simulink model "TLBO_2023"  (R2023b)
settings: Solver=ode45  StartTime=0.0  StopTime=6  MaxStep=1e-4  RelTol=1e-3  EnableMultiTasking=on
PreLoadFcn:
  | Ts_Power=1e-6;
  | Ts_Control=100e-6;
InitFcn:
  | Ts_Power=1e-6;
  | Ts_Control=100e-6;
  | Rtrans=0.142;
  | Xtrans=0.12e-6;
undefined symbols (not defined in the file): DiscIntNeverNeededParam, Ion, Lithium, sigbuilder_block
libraries: dspfdesign x80, spsSeriesRLCBranchLib x52, spsCurrentMeasurementLib x20, spsMeanLib x20, spsIdealSwitchLib x16, spsVoltageMeasurementLib x16, slpidlib x15, spsMosfetLib x14, dspindex x12, spsPWMGeneratorDCDCLib x10, spsGroundLib x10, spsBatteryLib x4
(part 2 of 4)

== system TLBO_2023/DC Load 1_2 ==
  note: DC Load Control
  1 : dspfdesign/Analog Filter Design  method=Butterworth  filttype=Lowpass  N=8  Wlo=pi*50  Whi=80  Rp=2  Rs=40
  2 : dspfdesign/Analog Filter Design  method=Butterworth  filttype=Lowpass  N=8  Wlo=pi*50  Whi=80  Rp=2  Rs=40
  Current Measurement3 : spsCurrentMeasurementLib/Current Measurement  PhasorSimulation=off  OutputType=Complex  PSBequivalent=0
  Demux : Demux
  Ideal Switch{,1..3} (4 alike) : spsIdealSwitchLib/Ideal Switch  Ron=0.001  Lon=0  IC=0  Rs=1e5  Cs=inf  Measurements=off
  Load Control : Subsystem  Tag=STV Subsys  LoadFcn=sigbuilder_block('load');  StartFcn=sigbuilder_block('start');  StopFcn=sigbuilder_block('stop');  ClipboardFcn=sigbuilder_block('clipboard');  mask(Sigbuilder block){tuvar=[0:10]}
      mask help: Sigbuilder GUI
      mask init:
      | if ~strcmp(get_param(bdroot(gcbh),'SimulationStatus'),'stopped') tuvar = sigbuilder_block('maskInit'); end
      settings: CopyFcn=sigbuilder_block('copy');  DeleteFcn=sigbuilder_block('delete');  ModelCloseFcn=sigbuilder_block('modelClose');  PreSaveFcn=sigbuilder_block('preSave');  PauseFcn=sigbuilder_block('pause')  ContinueFcn=sigbuilder_block('continue')  NameChangeFcn=sigbuilder_block('namechange');  OpenFcn=sigbuilder_block('open',[5.4 30 1141.2 522.6 ]);  CloseFcn=sigbuilder_block('close');
      mask Display: plot(0, 0, 100, 100,[2, 2, 32, 32, 2], [68, 8, 8, 68, 68],[32, 2], [38, 38], [32, 19, 2],[53, 60, 44], [32, 17, 17, 2],[16, 16, 31, 31]);txt = getActiveGroup(gcbh);text(2, 100, txt,'verticalAlignment', 'top');
  Mux3 : Mux
  Product : Product
  Scope1 : Scope  NumInputPorts=2
  Series RLC Branch5 : spsSeriesRLCBranchLib/Series RLC Branch  LConnTagsString=__new0  RConnTagsString=__new0  BranchType=R  Resistance=5  Inductance=1e-3  SetiL0=off  InitialCurrent=0  Capacitance=1000e-6  Setx0=off  InitialVoltage=0  Measurements=None
  Series RLC Branch6 : spsSeriesRLCBranchLib/Series RLC Branch  LConnTagsString=__new0  RConnTagsString=__new0  BranchType=R  Resistance=50  Inductance=1e-3  SetiL0=off  InitialCurrent=0  Capacitance=1000e-6  Setx0=off  InitialVoltage=0  Measurements=None
  Series RLC Branch7 : spsSeriesRLCBranchLib/Series RLC Branch  LConnTagsString=__new0  RConnTagsString=__new0  BranchType=R  Resistance=11.5  Inductance=1e-3  SetiL0=off  InitialCurrent=0  Capacitance=1000e-6  Setx0=off  InitialVoltage=0  Measurements=None
  Series RLC Branch8 : spsSeriesRLCBranchLib/Series RLC Branch  LConnTagsString=__new0  RConnTagsString=__new0  BranchType=R  Resistance=11.5  Inductance=1e-3  SetiL0=off  InitialCurrent=0  Capacitance=1000e-6  Setx0=off  InitialVoltage=0  Measurements=None
  Series RLC Branch9 : spsSeriesRLCBranchLib/Series RLC Branch  LConnTagsString=__new0  RConnTagsString=__new0  BranchType=R  Resistance=11.5  Inductance=1e-3  SetiL0=off  InitialCurrent=0  Capacitance=1000e-6  Setx0=off  InitialVoltage=0  Measurements=None
  Voltage Measurement2 : spsVoltageMeasurementLib/Voltage Measurement  PhasorSimulation=off  OutputType=Complex  PSBequivalent=0
  + : PMIOPort  Side=Left
  - : PMIOPort  Port=2  Side=Right
  tag scope: I_L2=global, P_L2=global, V_L2=global
  wires:
  Product/1 -> [P_L2]
  Mux3/1 -> Demux/1
  Load Control/1(S1) -> Mux3/1
  Load Control/2(S2) -> Mux3/2
  Load Control/4(S4) -> Mux3/4
  Voltage Measurement2/1 -> 1/1
  Current Measurement3/1 -> 2/1
  Load Control/3(S3) -> Mux3/3
  Demux/2 -> Ideal Switch1/1  "S3"
  Demux/4 -> Ideal Switch3/1  "S5"
  Demux/1 -> Ideal Switch/1  "S2"
  Demux/3 -> Ideal Switch2/1  "S4"
  1/1 -> Scope1/2, [V_L2], Product/2  "Load Voltage"
  2/1 -> Scope1/1, [I_L2], Product/1  "Load Current"
  connections:
  +/RConn1 -- Current Measurement3/LConn1
  Ideal Switch/RConn1 -- Series RLC Branch6/LConn1
  Ideal Switch2/RConn1 -- Series RLC Branch8/LConn1
  Ideal Switch3/RConn1 -- Series RLC Branch9/LConn1
  Ideal Switch1/RConn1 -- Series RLC Branch7/LConn1
  -/RConn1 -- Series RLC Branch7/RConn1 -- Series RLC Branch8/RConn1 -- Series RLC Branch9/RConn1 -- Series RLC Branch6/RConn1 -- Series RLC Branch5/RConn1 -- Voltage Measurement2/LConn2
  Series RLC Branch5/LConn1 -- Ideal Switch2/LConn1 -- Ideal Switch3/LConn1 -- Ideal Switch1/LConn1 -- Ideal Switch/LConn1 -- Voltage Measurement2/LConn1 -- Current Measurement3/RConn1

== system TLBO_2023/DC Load 1_4 ==
  note: DC Load Control
  note: Maximum Load Power = 230W
  1 : dspfdesign/Analog Filter Design  method=Butterworth  filttype=Lowpass  N=8  Wlo=pi*50  Whi=80  Rp=2  Rs=40
  2 : dspfdesign/Analog Filter Design  method=Butterworth  filttype=Lowpass  N=8  Wlo=pi*50  Whi=80  Rp=2  Rs=40
  Current Measurement3 : spsCurrentMeasurementLib/Current Measurement  PhasorSimulation=off  OutputType=Complex  PSBequivalent=0
  Demux : Demux
  Ideal Switch{,1..3} (4 alike) : spsIdealSwitchLib/Ideal Switch  Ron=0.001  Lon=0  IC=0  Rs=1e5  Cs=inf  Measurements=off
  Load Control : Subsystem  Tag=STV Subsys  LoadFcn=sigbuilder_block('load');  StartFcn=sigbuilder_block('start');  StopFcn=sigbuilder_block('stop');  ClipboardFcn=sigbuilder_block('clipboard');  mask(Sigbuilder block){tuvar=[0:10]}
      mask help: Sigbuilder GUI
      mask init:
      | if ~strcmp(get_param(bdroot(gcbh),'SimulationStatus'),'stopped') tuvar = sigbuilder_block('maskInit'); end
      settings: CopyFcn=sigbuilder_block('copy');  DeleteFcn=sigbuilder_block('delete');  ModelCloseFcn=sigbuilder_block('modelClose');  PreSaveFcn=sigbuilder_block('preSave');  PauseFcn=sigbuilder_block('pause')  ContinueFcn=sigbuilder_block('continue')  NameChangeFcn=sigbuilder_block('namechange');  OpenFcn=sigbuilder_block('open',[5.4 30 1141.2 522.6 ]);  CloseFcn=sigbuilder_block('close');
      mask Display: plot(0, 0, 100, 100,[2, 2, 32, 32, 2], [68, 8, 8, 68, 68],[32, 2], [38, 38], [32, 19, 2],[53, 60, 44], [32, 17, 17, 2],[16, 16, 31, 31]);txt = getActiveGroup(gcbh);text(2, 100, txt,'verticalAlignment', 'top');
  Mux3 : Mux
  Product : Product
  Scope1 : Scope  NumInputPorts=2
  Series RLC Branch5 : spsSeriesRLCBranchLib/Series RLC Branch  LConnTagsString=__new0  RConnTagsString=__new0  BranchType=R  Resistance=5  Inductance=1e-3  SetiL0=off  InitialCurrent=0  Capacitance=1000e-6  Setx0=off  InitialVoltage=0  Measurements=None
  Series RLC Branch{6..9} (4 alike) : spsSeriesRLCBranchLib/Series RLC Branch  LConnTagsString=__new0  RConnTagsString=__new0  BranchType=R  Resistance=50  Inductance=1e-3  SetiL0=off  InitialCurrent=0  Capacitance=1000e-6  Setx0=off  InitialVoltage=0  Measurements=None
  Voltage Measurement2 : spsVoltageMeasurementLib/Voltage Measurement  PhasorSimulation=off  OutputType=Complex  PSBequivalent=0
  + : PMIOPort  Side=Left
  - : PMIOPort  Port=2  Side=Left
  tag scope: I_L1=global, P_L1=global, V_L1=global
  wires:
  Demux/3 -> Ideal Switch2/1  "S4"
  Demux/1 -> Ideal Switch/1  "S2"
  Demux/4 -> Ideal Switch3/1  "S5"
  Demux/2 -> Ideal Switch1/1  "S3"
  Load Control/3(S3) -> Mux3/3
  Current Measurement3/1 -> 2/1
  1/1 -> [V_L1], Product/2, Scope1/2  "Load Voltage"
  Voltage Measurement2/1 -> 1/1
  2/1 -> [I_L1], Product/1, Scope1/1  "Load Current"
  Load Control/4(S4) -> Mux3/4
  Load Control/2(S2) -> Mux3/2
  Load Control/1(S1) -> Mux3/1
  Mux3/1 -> Demux/1
  Product/1 -> [P_L1]
  connections:
  Ideal Switch2/LConn1 -- Ideal Switch3/LConn1 -- Ideal Switch1/LConn1 -- Ideal Switch/LConn1 -- Series RLC Branch5/LConn1 -- Current Measurement3/RConn1 -- Voltage Measurement2/LConn1
  Series RLC Branch7/RConn1 -- Series RLC Branch9/RConn1 -- Series RLC Branch8/RConn1 -- Series RLC Branch6/RConn1 -- Series RLC Branch5/RConn1 -- -/RConn1 -- Voltage Measurement2/LConn2
  Ideal Switch1/RConn1 -- Series RLC Branch7/LConn1
  Ideal Switch3/RConn1 -- Series RLC Branch9/LConn1
  Ideal Switch2/RConn1 -- Series RLC Branch8/LConn1
  Ideal Switch/RConn1 -- Series RLC Branch6/LConn1
  +/RConn1 -- Current Measurement3/LConn1

== system TLBO_2023/DC Load 2_3 ==
  note: DC Load Control
  note: Maximum Load Power = 230W
  1 : dspfdesign/Analog Filter Design  method=Butterworth  filttype=Lowpass  N=8  Wlo=pi*50  Whi=80  Rp=2  Rs=40
  2 : dspfdesign/Analog Filter Design  method=Butterworth  filttype=Lowpass  N=8  Wlo=pi*50  Whi=80  Rp=2  Rs=40
  Current Measurement3 : spsCurrentMeasurementLib/Current Measurement  PhasorSimulation=off  OutputType=Complex  PSBequivalent=0
  Demux : Demux
  Ideal Switch{,1..3} (4 alike) : spsIdealSwitchLib/Ideal Switch  Ron=0.001  Lon=0  IC=0  Rs=1e5  Cs=inf  Measurements=off
  Load Control : Subsystem  Tag=STV Subsys  LoadFcn=sigbuilder_block('load');  StartFcn=sigbuilder_block('start');  StopFcn=sigbuilder_block('stop');  ClipboardFcn=sigbuilder_block('clipboard');  mask(Sigbuilder block){tuvar=[0:10]}
      mask help: Sigbuilder GUI
      mask init:
      | if ~strcmp(get_param(bdroot(gcbh),'SimulationStatus'),'stopped') tuvar = sigbuilder_block('maskInit'); end
      settings: CopyFcn=sigbuilder_block('copy');  DeleteFcn=sigbuilder_block('delete');  ModelCloseFcn=sigbuilder_block('modelClose');  PreSaveFcn=sigbuilder_block('preSave');  PauseFcn=sigbuilder_block('pause')  ContinueFcn=sigbuilder_block('continue')  NameChangeFcn=sigbuilder_block('namechange');  OpenFcn=sigbuilder_block('open',[5.4 30 1141.2 522.6 ]);  CloseFcn=sigbuilder_block('close');
      mask Display: plot(0, 0, 100, 100,[2, 2, 32, 32, 2], [68, 8, 8, 68, 68],[32, 2], [38, 38], [32, 19, 2],[53, 60, 44], [32, 17, 17, 2],[16, 16, 31, 31]);txt = getActiveGroup(gcbh);text(2, 100, txt,'verticalAlignment', 'top');
  Mux3 : Mux
  Product : Product
  Scope1 : Scope  NumInputPorts=2
  Series RLC Branch{5,7..9} (4 alike) : spsSeriesRLCBranchLib/Series RLC Branch  LConnTagsString=__new0  RConnTagsString=__new0  BranchType=R  Resistance=5  Inductance=1e-3  SetiL0=off  InitialCurrent=0  Capacitance=1000e-6  Setx0=off  InitialVoltage=0  Measurements=None
  Series RLC Branch6 : spsSeriesRLCBranchLib/Series RLC Branch  LConnTagsString=__new0  RConnTagsString=__new0  BranchType=R  Resistance=50  Inductance=1e-3  SetiL0=off  InitialCurrent=0  Capacitance=1000e-6  Setx0=off  InitialVoltage=0  Measurements=None
  Voltage Measurement2 : spsVoltageMeasurementLib/Voltage Measurement  PhasorSimulation=off  OutputType=Complex  PSBequivalent=0
  + : PMIOPort  Side=Left
  - : PMIOPort  Port=2  Side=Left
  tag scope: I_L3=global, P_L3=global, V_L3=global
  wires:
  Demux/3 -> Ideal Switch2/1  "S4"
  Demux/1 -> Ideal Switch/1  "S2"
  Demux/4 -> Ideal Switch3/1  "S5"
  Demux/2 -> Ideal Switch1/1  "S3"
  Load Control/3(S3) -> Mux3/3
  Current Measurement3/1 -> 2/1
  Voltage Measurement2/1 -> 1/1
  Load Control/4(S4) -> Mux3/4
  Load Control/2(S2) -> Mux3/2
  Load Control/1(S1) -> Mux3/1
  Mux3/1 -> Demux/1
  Product/1 -> [P_L3]
  1/1 -> [V_L3], Product/2, Scope1/2  "Load Voltage"
  2/1 -> [I_L3], Product/1, Scope1/1  "Load Current"
  connections:
  Current Measurement3/RConn1 -- Voltage Measurement2/LConn1 -- Ideal Switch/LConn1 -- Ideal Switch1/LConn1 -- Ideal Switch3/LConn1 -- Ideal Switch2/LConn1 -- Series RLC Branch5/LConn1
  Voltage Measurement2/LConn2 -- Series RLC Branch5/RConn1 -- Series RLC Branch6/RConn1 -- Series RLC Branch9/RConn1 -- Series RLC Branch8/RConn1 -- Series RLC Branch7/RConn1 -- -/RConn1
  Ideal Switch1/RConn1 -- Series RLC Branch7/LConn1
  Ideal Switch3/RConn1 -- Series RLC Branch9/LConn1
  Ideal Switch2/RConn1 -- Series RLC Branch8/LConn1
  Ideal Switch/RConn1 -- Series RLC Branch6/LConn1
  +/RConn1 -- Current Measurement3/LConn1

== system TLBO_2023/DC Load 3_4 ==
  note: DC Load Control
  1 : dspfdesign/Analog Filter Design  method=Butterworth  filttype=Lowpass  N=8  Wlo=pi*50  Whi=80  Rp=2  Rs=40
  2 : dspfdesign/Analog Filter Design  method=Butterworth  filttype=Lowpass  N=8  Wlo=pi*50  Whi=80  Rp=2  Rs=40
  Current Measurement3 : spsCurrentMeasurementLib/Current Measurement  PhasorSimulation=off  OutputType=Complex  PSBequivalent=0
  Demux : Demux
  Ideal Switch{,1..3} (4 alike) : spsIdealSwitchLib/Ideal Switch  Ron=0.001  Lon=0  IC=0  Rs=1e5  Cs=inf  Measurements=off
  Load Control : Subsystem  Tag=STV Subsys  LoadFcn=sigbuilder_block('load');  StartFcn=sigbuilder_block('start');  StopFcn=sigbuilder_block('stop');  ClipboardFcn=sigbuilder_block('clipboard');  mask(Sigbuilder block){tuvar=[0:10]}
      mask help: Sigbuilder GUI
      mask init:
      | if ~strcmp(get_param(bdroot(gcbh),'SimulationStatus'),'stopped') tuvar = sigbuilder_block('maskInit'); end
      settings: CopyFcn=sigbuilder_block('copy');  DeleteFcn=sigbuilder_block('delete');  ModelCloseFcn=sigbuilder_block('modelClose');  PreSaveFcn=sigbuilder_block('preSave');  PauseFcn=sigbuilder_block('pause')  ContinueFcn=sigbuilder_block('continue')  NameChangeFcn=sigbuilder_block('namechange');  OpenFcn=sigbuilder_block('open',[5.4 30 1141.2 522.6 ]);  CloseFcn=sigbuilder_block('close');
      mask Display: plot(0, 0, 100, 100,[2, 2, 32, 32, 2], [68, 8, 8, 68, 68],[32, 2], [38, 38], [32, 19, 2],[53, 60, 44], [32, 17, 17, 2],[16, 16, 31, 31]);txt = getActiveGroup(gcbh);text(2, 100, txt,'verticalAlignment', 'top');
  Mux3 : Mux
  Product : Product
  Scope1 : Scope  NumInputPorts=2
  Series RLC Branch5 : spsSeriesRLCBranchLib/Series RLC Branch  LConnTagsString=__new0  RConnTagsString=__new0  BranchType=R  Resistance=5  Inductance=1e-3  SetiL0=off  InitialCurrent=0  Capacitance=1000e-6  Setx0=off  InitialVoltage=0  Measurements=None
  Series RLC Branch6 : spsSeriesRLCBranchLib/Series RLC Branch  LConnTagsString=__new0  RConnTagsString=__new0  BranchType=R  Resistance=50  Inductance=1e-3  SetiL0=off  InitialCurrent=0  Capacitance=1000e-6  Setx0=off  InitialVoltage=0  Measurements=None
  Series RLC Branch7 : spsSeriesRLCBranchLib/Series RLC Branch  LConnTagsString=__new0  RConnTagsString=__new0  BranchType=R  Resistance=11.5  Inductance=1e-3  SetiL0=off  InitialCurrent=0  Capacitance=1000e-6  Setx0=off  InitialVoltage=0  Measurements=None
  Series RLC Branch8 : spsSeriesRLCBranchLib/Series RLC Branch  LConnTagsString=__new0  RConnTagsString=__new0  BranchType=R  Resistance=11.5  Inductance=1e-3  SetiL0=off  InitialCurrent=0  Capacitance=1000e-6  Setx0=off  InitialVoltage=0  Measurements=None
  Series RLC Branch9 : spsSeriesRLCBranchLib/Series RLC Branch  LConnTagsString=__new0  RConnTagsString=__new0  BranchType=R  Resistance=11.5  Inductance=1e-3  SetiL0=off  InitialCurrent=0  Capacitance=1000e-6  Setx0=off  InitialVoltage=0  Measurements=None
  Voltage Measurement2 : spsVoltageMeasurementLib/Voltage Measurement  PhasorSimulation=off  OutputType=Complex  PSBequivalent=0
  + : PMIOPort  Side=Left
  - : PMIOPort  Port=2  Side=Right
  tag scope: I_L4=global, P_L4=global, V_L4=global
  wires:
  Product/1 -> [P_L4]
  Mux3/1 -> Demux/1
  Load Control/1(S1) -> Mux3/1
  Load Control/2(S2) -> Mux3/2
  Load Control/4(S4) -> Mux3/4
  Voltage Measurement2/1 -> 1/1
  Current Measurement3/1 -> 2/1
  Load Control/3(S3) -> Mux3/3
  Demux/2 -> Ideal Switch1/1  "S3"
  Demux/4 -> Ideal Switch3/1  "S5"
  Demux/1 -> Ideal Switch/1  "S2"
  Demux/3 -> Ideal Switch2/1  "S4"
  1/1 -> Scope1/2, [V_L4], Product/2  "Load Voltage"
  2/1 -> Scope1/1, [I_L4], Product/1  "Load Current"
  connections:
  +/RConn1 -- Current Measurement3/LConn1
  Ideal Switch/RConn1 -- Series RLC Branch6/LConn1
  Ideal Switch2/RConn1 -- Series RLC Branch8/LConn1
  Ideal Switch3/RConn1 -- Series RLC Branch9/LConn1
  Ideal Switch1/RConn1 -- Series RLC Branch7/LConn1
  -/RConn1 -- Series RLC Branch7/RConn1 -- Series RLC Branch8/RConn1 -- Series RLC Branch9/RConn1 -- Series RLC Branch6/RConn1 -- Series RLC Branch5/RConn1 -- Voltage Measurement2/LConn2
  Series RLC Branch5/LConn1 -- Ideal Switch2/LConn1 -- Ideal Switch3/LConn1 -- Ideal Switch1/LConn1 -- Ideal Switch/LConn1 -- Voltage Measurement2/LConn1 -- Current Measurement3/RConn1

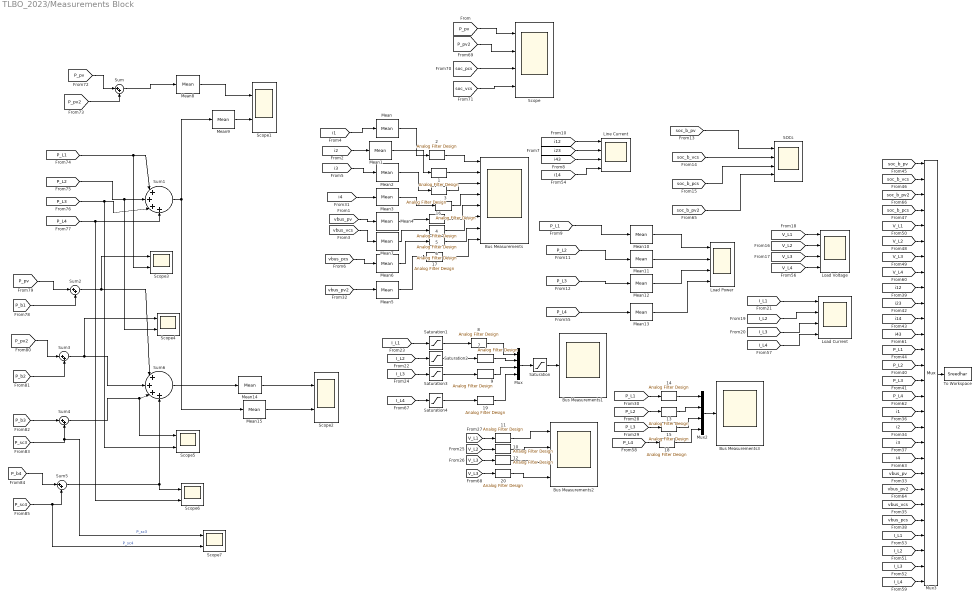
== system TLBO_2023/Measurements Block ==
  {1..20} (20 alike) : dspfdesign/Analog Filter Design  method=Butterworth  filttype=Lowpass  N=8  Wlo=pi*50  Whi=80  Rp=2  Rs=40
  Bus Measurements : Scope  NumInputPorts=8
  Bus Measurements1 : Scope
  Bus Measurements2 : Scope  NumInputPorts=4
  Bus Measurements3 : Scope
  Line Current : Scope  NumInputPorts=4
  Load Current : Scope  NumInputPorts=4
  Load Power : Scope  NumInputPorts=4
  Load Voltage : Scope  NumInputPorts=4
  Mean{,1..15} (16 alike) : spsMeanLib/Mean  Freq=10  Vinit=0  Ts=0
  Mux : Mux
  Mux2 : Mux
  Mux3 : Mux  Inputs=28
  SOCs : Scope  NumInputPorts=4
  Saturation{,1..4} (5 alike) : Saturate  UpperLimit=50  LowerLimit=0
  Scope : Scope  NumInputPorts=4
  Scope{1..7} (7 alike) : Scope  NumInputPorts=2
  Sum{,2..5} (5 alike) : Sum  Inputs=|++
  Sum1 : Sum  Inputs=|++++
  Sum6 : Sum  Inputs=|++++
  To Workspace : ToWorkspace  VariableName=Sreedhar  SampleTime=-1
  wires:
  [i12] -> Line Current/1
  [i23] -> Line Current/2
  [i43] -> Line Current/3
  [soc_b_pv] -> SOCs/1
  [soc_b_vcs] -> SOCs/2
  [soc_b_pcs] -> SOCs/3
  [V_L1] -> Load Voltage/1
  [V_L2] -> Load Voltage/2
  [V_L3] -> Load Voltage/3
  [I_L1] -> Load Current/1
  [I_L2] -> Load Current/2
  [I_L3] -> Load Current/3
  2/1 -> Bus Measurements/1
  1/1 -> Bus Measurements/2
  3/1 -> Bus Measurements/3
  9/1 -> Mux/3
  7/1 -> Mux/2
  8/1 -> Mux/1
  11/1 -> Bus Measurements2/1
  [V_L1] -> 11/1
  [V_L2] -> 10/1
  [V_L3] -> 12/1
  10/1 -> Bus Measurements2/2
  12/1 -> Bus Measurements2/3
  Mux2/1 -> Bus Measurements3/1
  14/1 -> Mux2/1
  13/1 -> Mux2/2
  15/1 -> Mux2/3
  [P_L1] -> 14/1
  [P_L2] -> 13/1
  [P_L3] -> 15/1
  Mux/1 -> Saturation/1
  Saturation/1 -> Bus Measurements1/1
  [I_L1] -> Saturation1/1
  Saturation1/1 -> 8/1
  [I_L2] -> Saturation2/1
  Saturation2/1 -> 7/1
  [I_L3] -> Saturation3/1
  Saturation3/1 -> 9/1
  Mux3/1 -> To Workspace/1
  [V_L1] -> Mux3/5
  [soc_b_pcs] -> Mux3/4
  [soc_b_vcs] -> Mux3/2
  [soc_b_pv] -> Mux3/1
  6/1 -> Bus Measurements/7
  5/1 -> Bus Measurements/6
  4/1 -> Bus Measurements/5
  16/1 -> Bus Measurements/4
  17/1 -> Bus Measurements/8
  [i14] -> Line Current/4
  [V_L4] -> Load Voltage/4
  [I_L4] -> Load Current/4
  [P_L4] -> 18/1
  18/1 -> Mux2/4
  [V_L2] -> Mux3/6
  [V_L3] -> Mux3/7
  [V_L4] -> Mux3/8
  [i12] -> Mux3/9
  [i23] -> Mux3/10
  [i14] -> Mux3/11
  [i43] -> Mux3/12
  [P_L1] -> Mux3/13
  [P_L2] -> Mux3/14
  [P_L3] -> Mux3/15
  [P_L4] -> Mux3/16
  [i1] -> Mux3/17
  [i2] -> Mux3/18
  [i3] -> Mux3/19
  [i4] -> Mux3/20
  [vbus_pv] -> Mux3/21
  [vbus_pv2] -> Mux3/22
  [vbus_vcs] -> Mux3/23
  [vbus_pcs] -> Mux3/24
  [I_L1] -> Mux3/25
  [I_L2] -> Mux3/26
  [I_L3] -> Mux3/27
  [I_L4] -> Mux3/28
  [soc_b_pv2] -> SOCs/4
  [soc_b_pv2] -> Mux3/3
  [I_L4] -> Saturation4/1
  Saturation4/1 -> 19/1
  19/1 -> Mux/4
  [V_L3] -> 20/1
  20/1 -> Bus Measurements2/4
  [P_pv] -> Scope/1
  [P_pv2] -> Scope/2
  [soc_pcs] -> Scope/3
  [soc_vcs] -> Scope/4
  [P_pv] -> Sum/1
  [P_pv2] -> Sum/2
  [P_L1] -> Scope3/2, Sum1/1
  [P_L2] -> Scope4/2, Sum1/2
  [P_L3] -> Scope5/2, Sum1/3
  [P_L4] -> Scope6/2, Sum1/4
  Sum1/1 -> Mean9/1, Mean15/1
  [P_pv] -> Sum2/1
  [P_b1] -> Sum2/2
  [P_pv2] -> Sum3/1
  [P_b2] -> Sum3/2
  [P_b3] -> Sum4/1
  [P_sc3] -> Scope7/1, Sum4/2  "P_sc3"
  [P_b4] -> Sum5/1
  [P_sc4] -> Scope7/2, Sum5/2  "P_sc4"
  Sum2/1 -> Scope3/1, Sum6/1
  Sum3/1 -> Scope4/1, Sum6/2
  Sum4/1 -> Scope5/1, Sum6/3
  Sum5/1 -> Sum6/4, Scope6/1
  Sum6/1 -> Mean14/1
  [i1] -> Mean/1
  Mean/1 -> 2/1
  [i2] -> Mean1/1
  Mean1/1 -> 1/1
  [i3] -> Mean2/1
  Mean2/1 -> 3/1
  [i4] -> Mean3/1
  Mean3/1 -> 16/1
  [vbus_pv] -> Mean4/1
  Mean4/1 -> 4/1
  [vbus_pv2] -> Mean5/1
  Mean5/1 -> 17/1
  [vbus_pcs] -> Mean6/1
  Mean6/1 -> 6/1
  [vbus_vcs] -> Mean7/1
  Mean7/1 -> 5/1
  Sum/1 -> Mean8/1
  Mean8/1 -> Scope1/1
  Mean9/1 -> Scope1/2
  [P_L1] -> Mean10/1
  Mean10/1 -> Load Power/1
  [P_L2] -> Mean11/1
  Mean11/1 -> Load Power/2
  [P_L3] -> Mean12/1
  Mean12/1 -> Load Power/3
  [P_L4] -> Mean13/1
  Mean13/1 -> Load Power/4
  Mean14/1 -> Scope2/1
  Mean15/1 -> Scope2/2

== system TLBO_2023/Source1 ==
  Battery Storage : Subsystem
  P_b : Display
      settings: Format=bank  Decimation=1000
  P_pv : Display
      settings: Format=bank  Decimation=1000
  R1 : spsSeriesRLCBranchLib/Series RLC Branch  LConnTagsString=__new0  RConnTagsString=__new0  BranchType=R  Resistance=0.2  Inductance=1e-3  SetiL0=off  InitialCurrent=0  Capacitance=220e-6  Setx0=off  InitialVoltage=0  Measurements=None
  R2 : spsSeriesRLCBranchLib/Series RLC Branch  LConnTagsString=__new0  RConnTagsString=__new0  BranchType=R  Resistance=0.2  Inductance=1e-3  SetiL0=off  InitialCurrent=0  Capacitance=220e-6  Setx0=off  InitialVoltage=0  Measurements=None
  Rooftop Solar System : Subsystem
  SOC_b : Display
      settings: Format=bank  Decimation=1000
  + : PMIOPort  Side=Right
  - : PMIOPort  Port=2  Side=Right
  tag scope: P_b1=global, P_pv=global, soc_pv=global
  wires:
  Battery Storage/2(Power) -> [P_b1], P_b/1
  Battery Storage/1(SOC) -> [soc_pv], SOC_b/1
  Rooftop Solar System/1(Power) -> [P_pv], P_pv/1
  connections:
  R1/LConn1 -- +/RConn1 -- R2/LConn1
  R1/RConn1 -- Rooftop Solar System/RConn1
  R2/RConn1 -- Battery Storage/RConn1
  Rooftop Solar System/RConn2 -- -/RConn1 -- Battery Storage/RConn2

== system TLBO_2023/Source2 ==
  Battery Storage : Subsystem
  P_b : Display
      settings: Format=bank  Decimation=1000
  P_pv : Display
      settings: Format=bank  Decimation=1000
  R1 : spsSeriesRLCBranchLib/Series RLC Branch  LConnTagsString=__new0  RConnTagsString=__new0  BranchType=R  Resistance=0.2  Inductance=1e-3  SetiL0=off  InitialCurrent=0  Capacitance=220e-6  Setx0=off  InitialVoltage=0  Measurements=None
  R2 : spsSeriesRLCBranchLib/Series RLC Branch  LConnTagsString=__new0  RConnTagsString=__new0  BranchType=R  Resistance=0.2  Inductance=1e-3  SetiL0=off  InitialCurrent=0  Capacitance=220e-6  Setx0=off  InitialVoltage=0  Measurements=None
  Rooftop Solar System : Subsystem
  SOC_b : Display
      settings: Format=bank  Decimation=1000
  + : PMIOPort  Side=Right
  - : PMIOPort  Port=2  Side=Right
  tag scope: P_b2=global, P_pv2=global, soc_pv2=global
  wires:
  Battery Storage/2(Power) -> [P_b2], P_b/1
  Battery Storage/1(SOC) -> [soc_pv2], SOC_b/1
  Rooftop Solar System/1(Power) -> [P_pv2], P_pv/1
  connections:
  R1/LConn1 -- +/RConn1 -- R2/LConn1
  R1/RConn1 -- Rooftop Solar System/RConn1
  R2/RConn1 -- Battery Storage/RConn1
  Rooftop Solar System/RConn2 -- -/RConn1 -- Battery Storage/RConn2

== system TLBO_2023/Source3 ==
  Battery Storage : Subsystem
  P_pcs : Display
      settings: Format=bank  Decimation=1000
  P_sc_pcs : Display
      settings: Format=bank  Decimation=1000
  R1 : spsSeriesRLCBranchLib/Series RLC Branch  LConnTagsString=__new0  RConnTagsString=__new0  BranchType=R  Resistance=0.2  Inductance=1e-3  SetiL0=off  InitialCurrent=0  Capacitance=220e-6  Setx0=off  InitialVoltage=0  Measurements=None
  R2 : spsSeriesRLCBranchLib/Series RLC Branch  LConnTagsString=__new0  RConnTagsString=__new0  BranchType=R  Resistance=0.2  Inductance=1e-3  SetiL0=off  InitialCurrent=0  Capacitance=220e-6  Setx0=off  InitialVoltage=0  Measurements=None
  SOC_pcs : Display
      settings: Format=bank  Decimation=1000
  SOC_sc_pcs : Display
      settings: Format=bank  Decimation=1000
  Scope : Scope  NumInputPorts=2
  Super Capacitor : Subsystem
  + : PMIOPort  Side=Right
  - : PMIOPort  Port=2  Side=Left
  tag scope: P_b3=global, P_sc3=global, soc_pcs=global, soc_sc_pcs=global
  wires:
  Battery Storage/1(SOC) -> SOC_pcs/1, [soc_pcs]
  Battery Storage/2(Power) -> [P_b3], P_pcs/1
  Super Capacitor/1(SOC) -> [soc_sc_pcs], Scope/1, SOC_sc_pcs/1
  Super Capacitor/2(Power) -> [P_sc3], Scope/2, P_sc_pcs/1
  connections:
  Battery Storage/RConn2 -- Super Capacitor/RConn2 -- -/RConn1
  R2/RConn1 -- Battery Storage/RConn1
  R2/LConn1 -- R1/LConn1 -- +/RConn1
  Super Capacitor/RConn1 -- R1/RConn1

== system TLBO_2023/Source4 ==
  Battery Storage : Subsystem
  P_sc_vcs : Display
      settings: Format=bank  Decimation=1000
  P_vcs : Display
      settings: Format=bank  Decimation=1000
  R1 : spsSeriesRLCBranchLib/Series RLC Branch  LConnTagsString=__new0  RConnTagsString=__new0  BranchType=R  Resistance=0.2  Inductance=1e-3  SetiL0=off  InitialCurrent=0  Capacitance=220e-6  Setx0=off  InitialVoltage=0  Measurements=None
  R2 : spsSeriesRLCBranchLib/Series RLC Branch  LConnTagsString=__new0  RConnTagsString=__new0  BranchType=R  Resistance=0.2  Inductance=1e-3  SetiL0=off  InitialCurrent=0  Capacitance=220e-6  Setx0=off  InitialVoltage=0  Measurements=None
  SOC_sc_vcs : Display
      settings: Format=bank  Decimation=1000
  SOC_vcs : Display
      settings: Format=bank  Decimation=1000
  Scope5 : Scope  NumInputPorts=2
  Super Capacitor : Subsystem
  + : PMIOPort  Side=Right
  - : PMIOPort  Port=2  Side=Right
  tag scope: P_b4=global, P_sc4=global, Soc_sc_vcs=global, soc_vcs=global
  wires:
  Battery Storage/2(Power) -> [P_b4], P_vcs/1
  Battery Storage/1(SOC) -> [soc_vcs], SOC_vcs/1
  Super Capacitor/1(SOC) -> [Soc_sc_vcs], Scope5/1, SOC_sc_vcs/1
  Super Capacitor/2(Power) -> [P_sc4], Scope5/2, P_sc_vcs/1
  connections:
  +/RConn1 -- R1/LConn1 -- R2/LConn1
  R2/RConn1 -- Battery Storage/RConn1
  Battery Storage/RConn2 -- Super Capacitor/RConn2 -- -/RConn1
  Super Capacitor/RConn1 -- R1/RConn1

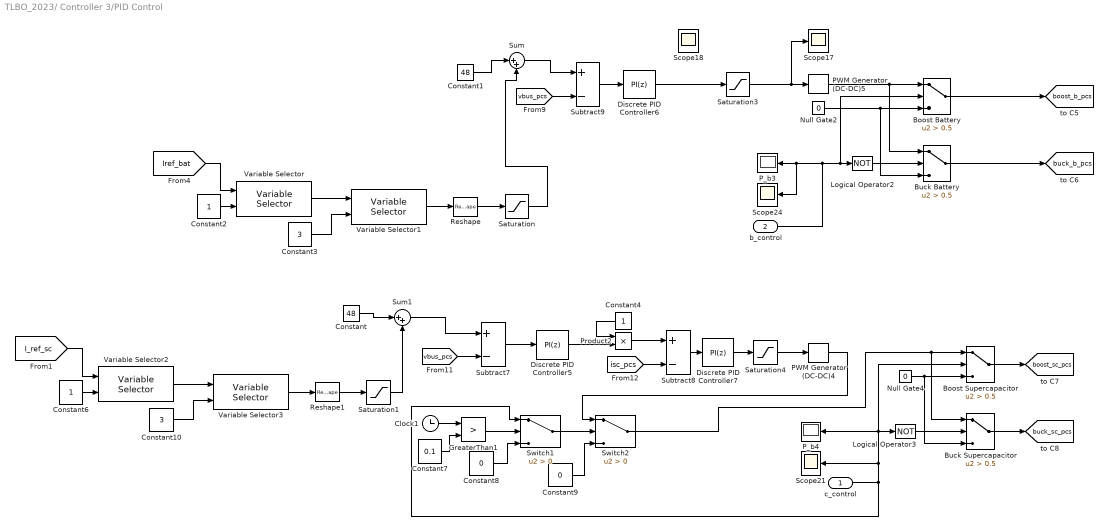
== system TLBO_2023/ Controller 3/PID Control ==
  c_control : Inport
  b_control : Inport  Port=2
  Boost Battery : Switch  Criteria=u2 > Threshold  Threshold=0.5  SaturateOnIntegerOverflow=off  InputSameDT=off
  Boost Supercapacitor : Switch  Criteria=u2 > Threshold  Threshold=0.5  SaturateOnIntegerOverflow=off  InputSameDT=off
  Buck Battery : Switch  Criteria=u2 > Threshold  Threshold=0.5  SaturateOnIntegerOverflow=off  InputSameDT=off
  Buck Supercapacitor : Switch  Criteria=u2 > Threshold  Threshold=0.5  SaturateOnIntegerOverflow=off  InputSameDT=off
  Clock1 : Clock
  Constant : Constant  Value=48
  Constant1 : Constant  Value=48
  Constant10 : Constant  Value=3
  Constant2 : Constant
  Constant3 : Constant  Value=3
  Constant4 : Constant
  Constant6 : Constant
  Constant7 : Constant  Value=0.1
  Constant8 : Constant  Value=0
  Constant9 : Constant  Value=0
  Discrete PID Controller5 : slpidlib/PID Controller  Controller=PI  Form=Parallel  TimeDomain=Discrete-time  UseExternalTs=off  SampleTime=-1  IntegratorMethod=Forward Euler  FilterMethod=Forward Euler  ControllerParametersSource=internal  P=0  I=4  UseKiTs=off  D=1  N=100  UseFilter=on  TunerSelectOption=Transfer Function Based (PID Tuner App)  InitialConditionSource=internal  InitialConditionForIntegrator=0  InitialConditionForFilter=0  DifferentiatorICPrevScaledInput=0  ExternalReset=none  TrackingMode=off  Kt=1  LimitOutput=off  SatLimitsSource=internal  UpperSaturationLimit=inf  LowerSaturationLimit=-inf  LinearizeAsGain=off  AntiWindupMode=none  Kb=1  LimitIntegrator=off  UpperIntegratorSaturationLimit=inf  LowerIntegratorSaturationLimit=-inf  POutMin=[]  POutMax=[]  IOutMin=[]  IOutMax=[]  DOutMin=[]  DOutMax=[]  NOutMin=[]  NOutMax=[]  SumOutMin=[]  SumOutMax=[]  SaturationOutMin=[]  SaturationOutMax=[]  PParamMin=[]  PParamMax=[]  IParamMin=[]  IParamMax=[]  DParamMin=[]  DParamMax=[]  NParamMin=[]  NParamMax=[]  KbParamMin=[]  KbParamMax=[]  KtParamMin=[]  KtParamMax=[]  KbOutMin=[]  KbOutMax=[]  KtOutMin=[]  KtOutMax=[]  IntegratorOutMin=[]  IntegratorOutMax=[]  FilterOutMin=[]  FilterOutMax=[]  SumI1OutMin=[]  SumI1OutMax=[]  SumI2OutMin=[]  SumI2OutMax=[]  SumI3OutMin=[]  SumI3OutMax=[]  SumI4OutMin=[]  SumI4OutMax=[]  SumDOutMin=[]  SumDOutMax=[]  DifferentiatorOutMin=[]  DifferentiatorOutMax=[]  FilterDiffOutCoefMin=[]  FilterDiffOutCoefMax=[]  ReciprocalOutMin=[]  ReciprocalOutMax=[]  SumDenOutMin=[]  SumDenOutMax=[]  SumNumOutMin=[]  SumNumOutMax=[]  DivideOutMin=[]  DivideOutMax=[]  UdiffTsProdOutMin=[]  UdiffTsProdOutMax=[]  NTsProdOutMin=[]  NTsProdOutMax=[]  UintegralTsProdOutMin=[]  UintegralTsProdOutMax=[]  UngainTsProdOutMin=[]  UngainTsProdOutMax=[]  ClampingZeroOutDataTypeStr=Inherit: Inherit via back propagation  ClampingZeroOutMin=[]  ClampingZeroOutMax=[]  FilterDenConstantOutDataTypeStr=Inherit: Inherit via back propagation  FilterDenConstantOutMin=[]  FilterDenConstantOutMax=[]  PCopyOutDataTypeStr=Inherit: Inherit via back propagation  PCopyOutMin=[]  PCopyOutMax=[]  NCopyOutDataTypeStr=Inherit: Inherit via back propagation  NCopyOutMin=[]  NCopyOutMax=[]  IntegratorContinuousStateAttributes=''  IntegratorStateMustResolveToSignalObject=off  IntegratorRTWStateStorageClass=Auto  FilterContinuousStateAttributes=''  FilterStateMustResolveToSignalObject=off  FilterRTWStateStorageClass=Auto  ParallelPVariant=InternalParameters  IdealPVariant=Disabled  IVariant=InternalParameters  DVariant=Disabled  IntegratorVariant=Discrete  SatVariant=Disabled  AWVariant=Passthrough  PCopyVariant=Disabled  TRVariant=Disabled  FdbkBlocksVariant=Forward  IdealPFdbkVariant=Disabled  SatFdbkVariant=Disabled  DerivativeFilterVariant=Disabled  NVariant=Disabled  NCopyVariant=Disabled_SignalSpec  FilterICVariant=Disabled  IntegratorICVariant=InternalICs  ExternalResetVariant=Disabled  TRSumVariant=Passthrough  SumFdbkVariant=Disabled  SumVariant=Sum_PI  TsampFilterVariant=InternalTs  TsampNgainVariant=Passthrough  TsampIntegralVariant=Disabled_SignalSpec  ExternalSaturationOutDataTypeStr=Inherit: Same as second input
  Discrete PID Controller6 : slpidlib/PID Controller  Controller=PI  Form=Parallel  TimeDomain=Discrete-time  UseExternalTs=off  SampleTime=-1  IntegratorMethod=Forward Euler  FilterMethod=Forward Euler  ControllerParametersSource=internal  P=0  I=1  UseKiTs=off  D=1  N=100  UseFilter=on  TunerSelectOption=Transfer Function Based (PID Tuner App)  InitialConditionSource=internal  InitialConditionForIntegrator=0  InitialConditionForFilter=0  DifferentiatorICPrevScaledInput=0  ExternalReset=none  TrackingMode=off  Kt=1  LimitOutput=off  SatLimitsSource=internal  UpperSaturationLimit=inf  LowerSaturationLimit=-inf  LinearizeAsGain=off  AntiWindupMode=none  Kb=1  LimitIntegrator=off  UpperIntegratorSaturationLimit=inf  LowerIntegratorSaturationLimit=-inf  POutMin=[]  POutMax=[]  IOutMin=[]  IOutMax=[]  DOutMin=[]  DOutMax=[]  NOutMin=[]  NOutMax=[]  SumOutMin=[]  SumOutMax=[]  SaturationOutMin=[]  SaturationOutMax=[]  PParamMin=[]  PParamMax=[]  IParamMin=[]  IParamMax=[]  DParamMin=[]  DParamMax=[]  NParamMin=[]  NParamMax=[]  KbParamMin=[]  KbParamMax=[]  KtParamMin=[]  KtParamMax=[]  KbOutMin=[]  KbOutMax=[]  KtOutMin=[]  KtOutMax=[]  IntegratorOutMin=[]  IntegratorOutMax=[]  FilterOutMin=[]  FilterOutMax=[]  SumI1OutMin=[]  SumI1OutMax=[]  SumI2OutMin=[]  SumI2OutMax=[]  SumI3OutMin=[]  SumI3OutMax=[]  SumI4OutMin=[]  SumI4OutMax=[]  SumDOutMin=[]  SumDOutMax=[]  DifferentiatorOutMin=[]  DifferentiatorOutMax=[]  FilterDiffOutCoefMin=[]  FilterDiffOutCoefMax=[]  ReciprocalOutMin=[]  ReciprocalOutMax=[]  SumDenOutMin=[]  SumDenOutMax=[]  SumNumOutMin=[]  SumNumOutMax=[]  DivideOutMin=[]  DivideOutMax=[]  UdiffTsProdOutMin=[]  UdiffTsProdOutMax=[]  NTsProdOutMin=[]  NTsProdOutMax=[]  UintegralTsProdOutMin=[]  UintegralTsProdOutMax=[]  UngainTsProdOutMin=[]  UngainTsProdOutMax=[]  ClampingZeroOutDataTypeStr=Inherit: Inherit via back propagation  ClampingZeroOutMin=[]  ClampingZeroOutMax=[]  FilterDenConstantOutDataTypeStr=Inherit: Inherit via back propagation  FilterDenConstantOutMin=[]  FilterDenConstantOutMax=[]  PCopyOutDataTypeStr=Inherit: Inherit via back propagation  PCopyOutMin=[]  PCopyOutMax=[]  NCopyOutDataTypeStr=Inherit: Inherit via back propagation  NCopyOutMin=[]  NCopyOutMax=[]  IntegratorContinuousStateAttributes=''  IntegratorStateMustResolveToSignalObject=off  IntegratorRTWStateStorageClass=Auto  FilterContinuousStateAttributes=''  FilterStateMustResolveToSignalObject=off  FilterRTWStateStorageClass=Auto  ParallelPVariant=InternalParameters  IdealPVariant=Disabled  IVariant=InternalParameters  DVariant=Disabled  IntegratorVariant=Discrete  SatVariant=Disabled  AWVariant=Passthrough  PCopyVariant=Disabled  TRVariant=Disabled  FdbkBlocksVariant=Forward  IdealPFdbkVariant=Disabled  SatFdbkVariant=Disabled  DerivativeFilterVariant=Disabled  NVariant=Disabled  NCopyVariant=Disabled_SignalSpec  FilterICVariant=Disabled  IntegratorICVariant=InternalICs  ExternalResetVariant=Disabled  TRSumVariant=Passthrough  SumFdbkVariant=Disabled  SumVariant=Sum_PI  TsampFilterVariant=InternalTs  TsampNgainVariant=Passthrough  TsampIntegralVariant=Disabled_SignalSpec  ExternalSaturationOutDataTypeStr=Inherit: Same as second input
  Discrete PID Controller7 : slpidlib/PID Controller  Controller=PI  Form=Parallel  TimeDomain=Discrete-time  UseExternalTs=off  SampleTime=-1  IntegratorMethod=Forward Euler  FilterMethod=Forward Euler  ControllerParametersSource=internal  P=0.2  I=4  UseKiTs=off  D=1  N=100  UseFilter=on  TunerSelectOption=Transfer Function Based (PID Tuner App)  InitialConditionSource=internal  InitialConditionForIntegrator=0  InitialConditionForFilter=0  DifferentiatorICPrevScaledInput=0  ExternalReset=none  TrackingMode=off  Kt=1  LimitOutput=off  SatLimitsSource=internal  UpperSaturationLimit=inf  LowerSaturationLimit=-inf  LinearizeAsGain=off  AntiWindupMode=none  Kb=1  LimitIntegrator=off  UpperIntegratorSaturationLimit=inf  LowerIntegratorSaturationLimit=-inf  POutMin=[]  POutMax=[]  IOutMin=[]  IOutMax=[]  DOutMin=[]  DOutMax=[]  NOutMin=[]  NOutMax=[]  SumOutMin=[]  SumOutMax=[]  SaturationOutMin=[]  SaturationOutMax=[]  PParamMin=[]  PParamMax=[]  IParamMin=[]  IParamMax=[]  DParamMin=[]  DParamMax=[]  NParamMin=[]  NParamMax=[]  KbParamMin=[]  KbParamMax=[]  KtParamMin=[]  KtParamMax=[]  KbOutMin=[]  KbOutMax=[]  KtOutMin=[]  KtOutMax=[]  IntegratorOutMin=[]  IntegratorOutMax=[]  FilterOutMin=[]  FilterOutMax=[]  SumI1OutMin=[]  SumI1OutMax=[]  SumI2OutMin=[]  SumI2OutMax=[]  SumI3OutMin=[]  SumI3OutMax=[]  SumI4OutMin=[]  SumI4OutMax=[]  SumDOutMin=[]  SumDOutMax=[]  DifferentiatorOutMin=[]  DifferentiatorOutMax=[]  FilterDiffOutCoefMin=[]  FilterDiffOutCoefMax=[]  ReciprocalOutMin=[]  ReciprocalOutMax=[]  SumDenOutMin=[]  SumDenOutMax=[]  SumNumOutMin=[]  SumNumOutMax=[]  DivideOutMin=[]  DivideOutMax=[]  UdiffTsProdOutMin=[]  UdiffTsProdOutMax=[]  NTsProdOutMin=[]  NTsProdOutMax=[]  UintegralTsProdOutMin=[]  UintegralTsProdOutMax=[]  UngainTsProdOutMin=[]  UngainTsProdOutMax=[]  ClampingZeroOutDataTypeStr=Inherit: Inherit via back propagation  ClampingZeroOutMin=[]  ClampingZeroOutMax=[]  FilterDenConstantOutDataTypeStr=Inherit: Inherit via back propagation  FilterDenConstantOutMin=[]  FilterDenConstantOutMax=[]  PCopyOutDataTypeStr=Inherit: Inherit via back propagation  PCopyOutMin=[]  PCopyOutMax=[]  NCopyOutDataTypeStr=Inherit: Inherit via back propagation  NCopyOutMin=[]  NCopyOutMax=[]  IntegratorContinuousStateAttributes=''  IntegratorStateMustResolveToSignalObject=off  IntegratorRTWStateStorageClass=Auto  FilterContinuousStateAttributes=''  FilterStateMustResolveToSignalObject=off  FilterRTWStateStorageClass=Auto  ParallelPVariant=InternalParameters  IdealPVariant=Disabled  IVariant=InternalParameters  DVariant=Disabled  IntegratorVariant=Discrete  SatVariant=Disabled  AWVariant=Passthrough  PCopyVariant=Disabled  TRVariant=Disabled  FdbkBlocksVariant=Forward  IdealPFdbkVariant=Disabled  SatFdbkVariant=Disabled  DerivativeFilterVariant=Disabled  NVariant=Disabled  NCopyVariant=Disabled_SignalSpec  FilterICVariant=Disabled  IntegratorICVariant=InternalICs  ExternalResetVariant=Disabled  TRSumVariant=Passthrough  SumFdbkVariant=Disabled  SumVariant=Sum_PI  TsampFilterVariant=InternalTs  TsampNgainVariant=Passthrough  TsampIntegralVariant=Disabled_SignalSpec  ExternalSaturationOutDataTypeStr=Inherit: Same as second input
  GreaterThan1 : RelationalOperator  Operator=>  OutDataTypeStr=boolean  RndMeth=Simplest  InputSameDT=off
  Logical Operator2 : Logic  Operator=NOT  AllPortsSameDT=off  OutDataTypeStr=boolean
  Logical Operator3 : Logic  Operator=NOT  AllPortsSameDT=off  OutDataTypeStr=boolean
  Null Gate2 : Constant  Value=0
  Null Gate4 : Constant  Value=0
  PWM Generator (DC-DC)4 : spsPWMGeneratorDCDCLib/PWM Generator (DC-DC)  Fsw=10e3  Ts=0
  PWM Generator (DC-DC)5 : spsPWMGeneratorDCDCLib/PWM Generator (DC-DC)  Fsw=10e3  Ts=0
  P_b3 : Display
      settings: Format=binary (Stored Integer)  Decimation=1000
  P_b4 : Display
      settings: Format=binary (Stored Integer)  Decimation=1000
  Product2 : Product
  Reshape : Reshape
  Reshape1 : Reshape
  Saturation : Saturate
  Saturation1 : Saturate
  Saturation3 : Saturate  UpperLimit=0.8  LowerLimit=0  ZeroCross=off
  Saturation4 : Saturate  UpperLimit=0.8  LowerLimit=0  ZeroCross=off
  Scope{17..18,21,24} (4 alike) : Scope
  Subtract7 : Sum  Inputs=+-
  Subtract8 : Sum  Inputs=+-
  Subtract9 : Sum  Inputs=+-
  Sum : Sum  Inputs=|++
  Sum1 : Sum  Inputs=|++
  Switch1 : Switch  Criteria=u2 > Threshold  SaturateOnIntegerOverflow=off  InputSameDT=off
  Switch2 : Switch  Criteria=u2 > Threshold  SaturateOnIntegerOverflow=off  InputSameDT=off
  Variable Selector : dspindex/Variable Selector  NumInputs=1  rowsOrCols=Rows  IdxMode=Variable  Elements=[1 3]  ZerOneIdxMode=One-based  errmode=Clip Index  FillMode=on  FillValues=0
  Variable Selector1 : dspindex/Variable Selector  NumInputs=1  rowsOrCols=Columns  IdxMode=Variable  Elements=[1 3]  ZerOneIdxMode=One-based  errmode=Clip Index  FillMode=on  FillValues=0
  Variable Selector2 : dspindex/Variable Selector  NumInputs=1  rowsOrCols=Rows  IdxMode=Variable  Elements=[1 3]  ZerOneIdxMode=One-based  errmode=Clip Index  FillMode=on  FillValues=0
  Variable Selector3 : dspindex/Variable Selector  NumInputs=1  rowsOrCols=Columns  IdxMode=Variable  Elements=[1 3]  ZerOneIdxMode=One-based  errmode=Clip Index  FillMode=on  FillValues=0
  tag scope: boost_b_pcs=global, boost_sc_pcs=global, buck_b_pcs=global, buck_sc_pcs=global
  wires:
  Buck Battery/1 -> [buck_b_pcs]
  Null Gate2/1 -> Boost Battery/3, Buck Battery/3
  b_control/1 -> Boost Battery/2, Logical Operator2/1, Scope24/1, P_b3/1
  Boost Battery/1 -> [boost_b_pcs]
  PWM Generator (DC-DC)5/1 -> Buck Battery/1, Boost Battery/1
  Logical Operator2/1 -> Buck Battery/2
  [vbus_pcs] -> Subtract9/2
  Buck Supercapacitor/1 -> [buck_sc_pcs]
  Null Gate4/1 -> Buck Supercapacitor/3, Boost Supercapacitor/3
  Boost Supercapacitor/1 -> [boost_sc_pcs]
  Logical Operator3/1 -> Buck Supercapacitor/2
  Subtract7/1 -> Discrete PID Controller5/1
  [vbus_pcs] -> Subtract7/2
  Saturation4/1 -> PWM Generator (DC-DC)4/1
  Saturation3/1 -> Scope17/1, PWM Generator (DC-DC)5/1
  [isc_pcs] -> Subtract8/2
  Product2/1 -> Subtract8/1
  Discrete PID Controller5/1 -> Product2/2
  Constant4/1 -> Product2/1
  Subtract8/1 -> Discrete PID Controller7/1
  Discrete PID Controller7/1 -> Saturation4/1
  [Iref_bat] -> Variable Selector/1
  Reshape/1 -> Saturation/1
  Variable Selector/1 -> Variable Selector1/1
  Constant2/1 -> Variable Selector/2
  Variable Selector1/1 -> Reshape/1
  Constant3/1 -> Variable Selector1/2
  Subtract9/1 -> Discrete PID Controller6/1
  Discrete PID Controller6/1 -> Saturation3/1
  Constant1/1 -> Sum/1
  Sum/1 -> Subtract9/1
  c_control/1 -> Switch1/1, Scope21/1, Logical Operator3/1, Boost Supercapacitor/2, P_b4/1
  GreaterThan1/1 -> Switch1/2
  Clock1/1 -> GreaterThan1/1
  Constant7/1 -> GreaterThan1/2
  Constant8/1 -> Switch1/3
  Switch1/1 -> Switch2/2
  Constant9/1 -> Switch2/3
  PWM Generator (DC-DC)4/1 -> Switch2/1
  Switch2/1 -> Buck Supercapacitor/1, Boost Supercapacitor/1
  Saturation/1 -> Sum/2
  [I_ref_sc] -> Variable Selector2/1
  Constant6/1 -> Variable Selector2/2
  Constant10/1 -> Variable Selector3/2
  Variable Selector3/1 -> Reshape1/1
  Variable Selector2/1 -> Variable Selector3/1
  Reshape1/1 -> Saturation1/1
  Saturation1/1 -> Sum1/2
  Constant/1 -> Sum1/1
  Sum1/1 -> Subtract7/1
